simulink model "Square_Timing_Recovery"  (Simulink 8.6)
settings: Solver=FixedStepDiscrete  StartTime=0  StopTime=inf  RelTol=1e-3
undefined symbols (not defined in the file): gcbh, magnitude, rcfiltgaincompat
libraries: commfilt2 x2, commchan3 x1, dspsigops x1, simulink x1, commdigbbndpm3 x1, commrandsrc2 x1, dspxfrm3 x1, dspobslib x1
CloseFcn:
  | rtwprivate ssgencode ModelCloseRequest Nyquist_Bedingungen
settings Model: Creator=schwall  LastModifiedBy=wunsch
settings DataIOCC: SaveOutput=off  SignalLogging=off  SaveTime=off
settings DebuggingCC: FcnCallInpInsideContextMsg=UseLocalSettings
settings SFSimCC: SimParseCustomCode=off
settings ConfigComp: CovSFcnEnable=off

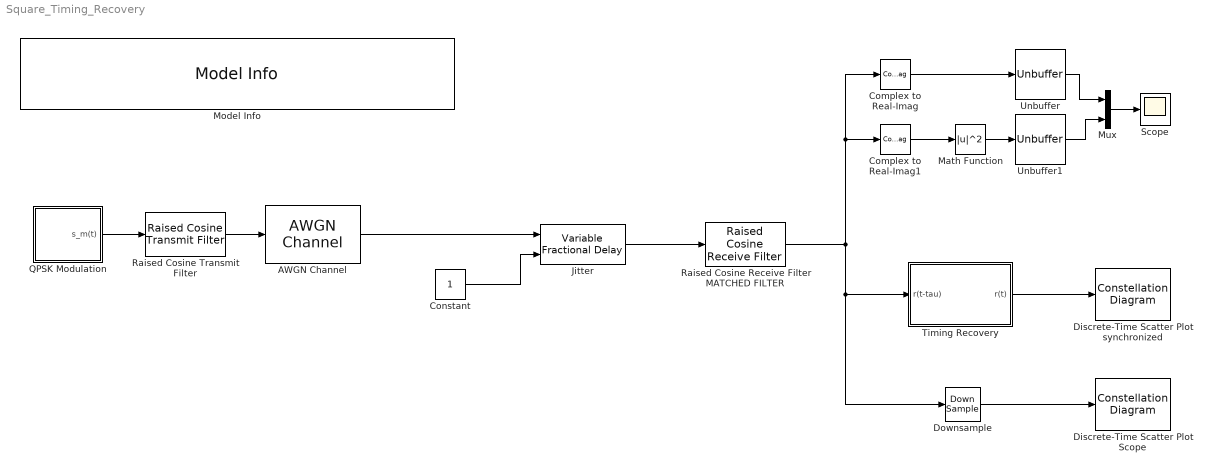
== system Square_Timing_Recovery ==
  AWGN Channel : commchan3/AWGN Channel  InputProcessing=Inherited (this choice will be removed - see release notes)  seed=67  noiseMode="Signal to noise ratio  (Es/No)"  EbNodB=10  EsNodB=100  SNRdB=100  bitsPerSym=1  Ps=1/8  Tsym=1/1000  variance=1
  Complex to Real-Imag : ComplexToRealImag  Output=Real
  Complex to Real-Imag1 : ComplexToRealImag  Output=Real
  Constant : Constant
  Discrete-Time Scatter Plot Scope : ConstellationDiagram  Tag=ScatterPlot
  Discrete-Time Scatter Plot synchronized : ConstellationDiagram  Tag=ScatterPlot
  Downsample : DownSample  N=8  InputProcessing=Inherited (this choice will be removed - see release notes)  smode=Force single rate  fmode=Maintain input frame rate
  Jitter : dspsigops/Variable Fractional Delay  mode=OBSOLETE  modeActive=Linear  dmax=100  InputProcessing=Columns as channels (frame based)  L=4  FarrowL=4  R=10  alpha=1  ic=0  fallbackFIR=Clip to the minimum value necessary for centered kernel  fallbackFarrow=Clip to the minimum value necessary for centered kernel  noDFT=off  roundingMode=Zero  overflowMode=off
  Math Function : Math  Operator=magnitude^2  SaturateOnIntegerOverflow=on
  Model Info : simulink/Model-Wide Utilities/Model Info  BlockCM=None  Frame=on  DisplayStringWithTags=|  HorizontalTextAlignment=Left  LeftAlignmentValue=0.02  SourceBlockDiagram=Square_Timing_Recovery  TagMaxNumber=20
      | Demo Square Timing Recovery
      | Vorlesung Nachrichtentechnik II
      | Institut fuer Nachrichtentechnik (CEL)
  Mux : Mux  Inputs=2
  QPSK Modulation : Subsystem
  Raised Cosine Receive Filter MATCHED FILTER : commfilt2/Raised Cosine Receive Filter  filtType=Square root  N=8  filtSpan=2*(4)  currentFiltSpan=2*(4)  D=4  R=1  sampMode=Mute  saveAsFlag=0  rateMode=Downsampling  downFactor=1  downOffset=0  framing=Maintain input frame rate  InputProcessing=Columns as channels (frame based)  checkGain=User-specified  filterGain=(1)*rcfiltgaincompat(gcbh)  checkCoeff=off  variableName=rcRxFilt  launchFVT=off  roundingMode=Floor  overflowMode=off
  Raised Cosine Transmit Filter : commfilt2/Raised Cosine Transmit Filter  filtType=Square root  filtSpan=2*(4)  currentFiltSpan=2*(4)  D=4  R=1  sampMode=Mute  saveAsFlag=0  N=8  framing=Maintain input frame rate  InputProcessing=Columns as channels (frame based)  checkGain=User-specified  filterGain=(1)*rcfiltgaincompat(gcbh)  checkCoeff=off  variableName=rcTxFilt  launchFVT=off  roundingMode=Floor  overflowMode=off
  Scope : Scope
  Timing Recovery : Subsystem
  Unbuffer : Unbuffer  SampleBasedProcessing=Same as frame based
  Unbuffer1 : Unbuffer  SampleBasedProcessing=Same as frame based
  wires:
  QPSK Modulation/1(s_m(t)) -> Raised Cosine Transmit Filter/1
  Downsample/1 -> Discrete-Time Scatter Plot Scope/1
  Raised Cosine Transmit Filter/1 -> AWGN Channel/1
  Raised Cosine Receive Filter MATCHED FILTER/1 -> Complex to Real-Imag1/1, Complex to Real-Imag/1, Downsample/1, Timing Recovery/1(r(t-tau))
  Timing Recovery/1(r(t)) -> Discrete-Time Scatter Plot synchronized/1
  Complex to Real-Imag/1 -> Unbuffer/1
  Complex to Real-Imag1/1 -> Math Function/1
  Math Function/1 -> Unbuffer1/1
  Unbuffer/1 -> Mux/1
  Mux/1 -> Scope/1
  Unbuffer1/1 -> Mux/2
  Constant/1 -> Jitter/2
  AWGN Channel/1 -> Jitter/1
  Jitter/1 -> Raised Cosine Receive Filter MATCHED FILTER/1

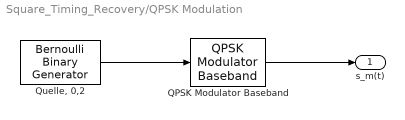
== system Square_Timing_Recovery/QPSK Modulation ==
  QPSK Modulator Baseband : commdigbbndpm3/QPSK Modulator Baseband  InType=Bit  Enc=Binary  Ph=pi/4  outDtype=double  outWordLen=16  outUDDataType=sfix(16)  outFracLenMode=Best precision  outFracLen=15
  "Quelle, 0,2" : commrandsrc2/Bernoulli Binary Generator  P=0.5  seed=61  Ts=1/1000/2  frameBased=on  sampPerFrame=128  orient=off  outDataType=double
  s_m(t) : Outport
  wires:
  "Quelle, 0,2"/1 -> QPSK Modulator Baseband/1
  QPSK Modulator Baseband/1 -> s_m(t)/1

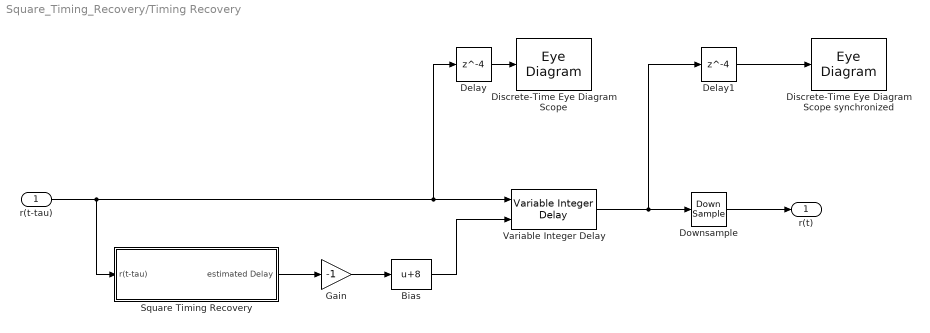
== system Square_Timing_Recovery/Timing Recovery ==
  r(t-tau) : Inport
  Bias : Bias  Bias=8
  Delay : Delay  DelayLength=4  InitialCondition=0  InputProcessing=Columns as channels (frame based)
  Delay1 : Delay  DelayLength=4  InitialCondition=0  InputProcessing=Columns as channels (frame based)
  Discrete-Time Eye Diagram Scope : EyeDiagram  Tag=EyeDiagram
  Discrete-Time Eye Diagram Scope synchronized : EyeDiagram  Tag=EyeDiagram
  Downsample : DownSample  N=8  InputProcessing=Inherited (this choice will be removed - see release notes)  smode=Force single rate  fmode=Maintain input frame rate
  Gain : Gain  Gain=-1
  Square Timing Recovery : Subsystem
  Variable Integer Delay : dspobslib/Variable Integer Delay  dmax=100  InputProcessing=Inherited (this choice will be removed - see release notes)  ic=0  noDFT=off
  r(t) : Outport
  wires:
  r(t-tau)/1 -> Square Timing Recovery/1(r(t-tau)), Delay/1, Variable Integer Delay/1
  Square Timing Recovery/1(estimated Delay) -> Gain/1
  Gain/1 -> Bias/1
  Bias/1 -> Variable Integer Delay/2
  Variable Integer Delay/1 -> Delay1/1, Downsample/1
  Downsample/1 -> r(t)/1
  Delay1/1 -> Discrete-Time Eye Diagram Scope synchronized/1
  Delay/1 -> Discrete-Time Eye Diagram Scope/1

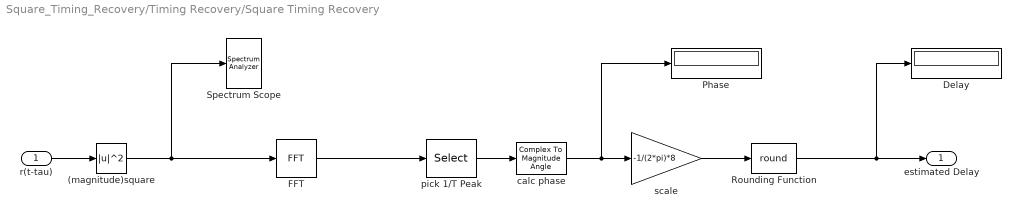
== system Square_Timing_Recovery/Timing Recovery/Square Timing Recovery ==
  r(t-tau) : Inport
  (magnitude)square : Math  Operator=magnitude^2  SaturateOnIntegerOverflow=on
  Delay : Display
  FFT : dspxfrm3/FFT  FFTImplementation=Auto  CompMethod=Table lookup  TableOpt=NEW  TableOptActive=Speed  BitRevOrder=off  Normalize=off  InheritFFTLength=on  FFTLength=64  WrapInput=on  roundingMode=Floor  overflowMode=off  firstCoeffDataTypeStr=Inherit: Same word length as input  firstCoeffLastDataTypeStr=Inherit: Same word length as input  outputMin=[]  outputMax=[]
  Phase : Display
  Rounding Function : Rounding  Operator=round
  Spectrum Scope : SpectrumAnalyzer
  calc phase : ComplexToMagnitudeAngle  Output=Angle
  pick 1/T Peak : Selector  InputPortWidth=512  IndexOptions=Index vector (dialog)  Indices=[65]  OutputSizes=1
  scale : Gain  Gain=-1/(2*pi)*8
  estimated Delay : Outport
  wires:
  (magnitude)square/1 -> FFT/1, Spectrum Scope/1
  FFT/1 -> pick 1/T Peak/1
  pick 1/T Peak/1 -> calc phase/1
  calc phase/1 -> scale/1, Phase/1
  scale/1 -> Rounding Function/1
  r(t-tau)/1 -> (magnitude)square/1
  Rounding Function/1 -> estimated Delay/1, Delay/1
